simulink library "sm_trackV_lib_belt_contact_internal_sets"  (R2026a)
settings: Solver=VariableStepAuto
undefined symbols (not defined in the file): A, B, L01, L02, L03, L04, L05, L06, L07, L08, L09, L1, L10, L11, L12, L13, L14, L15, L16, L17, L18, L19, L2, L20, L21, L22, L23, L24, L25, L26, L27, L28, L29, L3, L30, L31, L32, L33, L34, L35, L36, L37, L38, L39, L40, L41, L42, L43, L44, L45, P00, P01, P02, P03, P04, P05, P06, P07, P08, P09 ... (+59)
libraries: sm_trackV_lib_belt_contact x132, $bdroot x51
Description:
  | Copyright 2024-2026 The MathWorks, Inc.
settings Model: Creator=smiller  LastModifiedBy=smiller

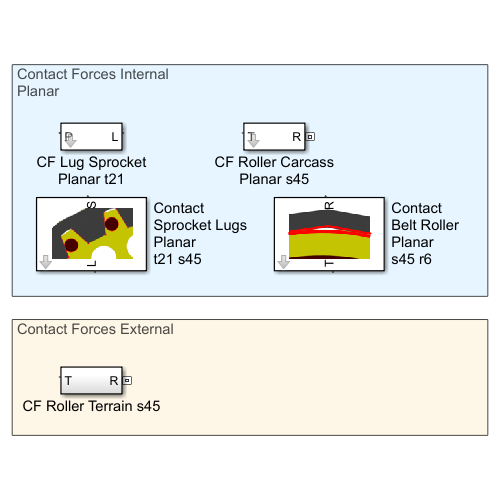
[thumbnail: Simulink's stored preview of the top-level diagram]
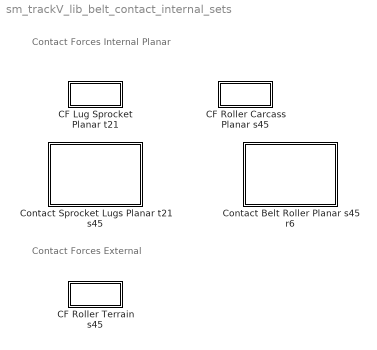
== system sm_trackV_lib_belt_contact_internal_sets ==
  note: Contact Forces External
  note: Contact Forces Internal
      | Planar
  CF Lug Sprocket Planar t21 : Subsystem  mask{K_SprocketLug=Trac.Contact.SprocketLug.K, B_SprocketLug=Trac.Contact.SprocketLug.B, TW_SprocketLug=Trac.Contact.SprocketLug.TW}
      mask prompts: K_SprocketLug "Normal Stiffness (N/m)"; B_SprocketLug "Normal Damping (N/(m/s))"; TW_SprocketLug "Normal Transition Width (m)"
  CF Roller Carcass Planar s45 : Subsystem  mask{K_Roller=Trac.Contact.Roller.K, B_Roller=Trac.Contact.Roller.B, TW_Roller=Trac.Contact.Roller.TW}
      mask prompts: K_Roller "Normal Stiffness (N/m)"; B_Roller "Normal Damping (N/(m/s))"; TW_Roller "Normal Transition Width (m)"
  CF Roller Terrain s45 : Subsystem
  Contact Belt Roller Planar s45 r6 : Subsystem  mask(Contact Force (Planar), Belt to 6 Rollers){K_SprocketRoller=Trac.Contact.SprocketRoller.K, B_SprocketRoller=Trac.Contact.SprocketRoller.B, TW_SprocketRoller=Trac.Contact.SprocketRoller.TW, K_IdlerFix=Trac.Contact.IdlerR.K, B_IdlerFix=Trac.Contact.IdlerR.B, TW_IdlerFix=Trac.Contact.IdlerR.TW, K_IdlerArm=Trac.Contact.IdlerF.K, B_IdlerArm=Trac.Contact.IdlerF.B, TW_IdlerArm=Trac.Contact.IdlerF.TW, K_Roller=Trac.Contact.Roller.K, B_Roller=Trac.Contact.Roller.B, TW_Roller=Trac.Contact.Roller.TW}
      mask prompts: K_SprocketRoller "Normal Stiffness (N/m)"; B_SprocketRoller "Normal Damping (N/(m/s))"; TW_SprocketRoller "Normal Transition Width (m)"; K_IdlerFix "Normal Stiffness (N/m)"; B_IdlerFix "Normal Damping (N/(m/s))"; TW_IdlerFix "Normal Transition Width (m)"; K_IdlerArm "Normal Stiffness (N/m)"; B_IdlerArm "Normal Damping (N/(m/s))"; TW_IdlerArm "Normal Transition Width (m)"; K_Roller "Normal Stiffness (N/m)"; B_Roller "Normal Damping (N/(m/s))"; TW_Roller "Normal Transition Width (m)"
      mask help: Models contact forces between entire belt (45 segments) and 6 rollers.
      mask TypeOptions K_SprocketRoller:
      | CF Roller
      | Sprocket/K_Roller
      mask TypeOptions B_SprocketRoller:
      | CF Roller
      | Sprocket/B_Roller
      mask TypeOptions TW_SprocketRoller:
      | CF Roller
      | Sprocket/TW_Roller
      mask TypeOptions K_IdlerFix:
      | CF Roller
      | Idler Fix/K_Roller
      mask TypeOptions B_IdlerFix:
      | CF Roller
      | Idler Fix/B_Roller
      mask TypeOptions TW_IdlerFix:
      | CF Roller
      | Idler Fix/TW_Roller
      mask TypeOptions K_IdlerArm:
      | CF Roller
      | Idler Arm/K_Roller
      mask TypeOptions B_IdlerArm:
      | CF Roller
      | Idler Arm/B_Roller
      mask TypeOptions TW_IdlerArm:
      | CF Roller
      | Idler Arm/TW_Roller
      mask TypeOptions K_Roller:
      | CF Roller
      | Roller L1/K_Roller | CF Roller
      | Roller L2/K_Roller | CF Roller
      | Roller L3/K_Roller
      mask TypeOptions B_Roller:
      | CF Roller
      | Roller L1/B_Roller | CF Roller
      | Roller L2/B_Roller | CF Roller
      | Roller L3/B_Roller
      mask TypeOptions TW_Roller:
      | CF Roller
      | Roller L1/TW_Roller | CF Roller
      | Roller L2/TW_Roller | CF Roller
      | Roller L3/TW_Roller
      mask DialogControl cont_contact_sprocketLug Prompt: Sprocket Roller
      mask DialogControl cont_contact_idlerFix Prompt: Idler Fixed
      mask DialogControl cont_contact_idlerArm Prompt: Idler Arm
      mask DialogControl cont_contact_rollerL Prompt: Lower Roller
      mask Display: image('sm_belt_cf_roller_carcass_IMAGE.png')
  Contact Sprocket Lugs Planar t21 s45 : Subsystem  mask(Contact Force (Planar), Belt to Sprocket){K_SprocketLug=Trac.Contact.SprocketLug.K, B_SprocketLug=Trac.Contact.SprocketLug.B, TW_SprocketLug=Trac.Contact.SprocketLug.TW}
      mask prompts: K_SprocketLug "Normal Stiffness (N/m)"; B_SprocketLug "Normal Damping (N/(m/s))"; TW_SprocketLug "Normal Transition Width (m)"
      mask help: Models contact forces between belt (45 lugs) and sprocket (21 pins).
      mask Display: image('sm_belt_cf_sprocket_lugs_IMAGE.png');

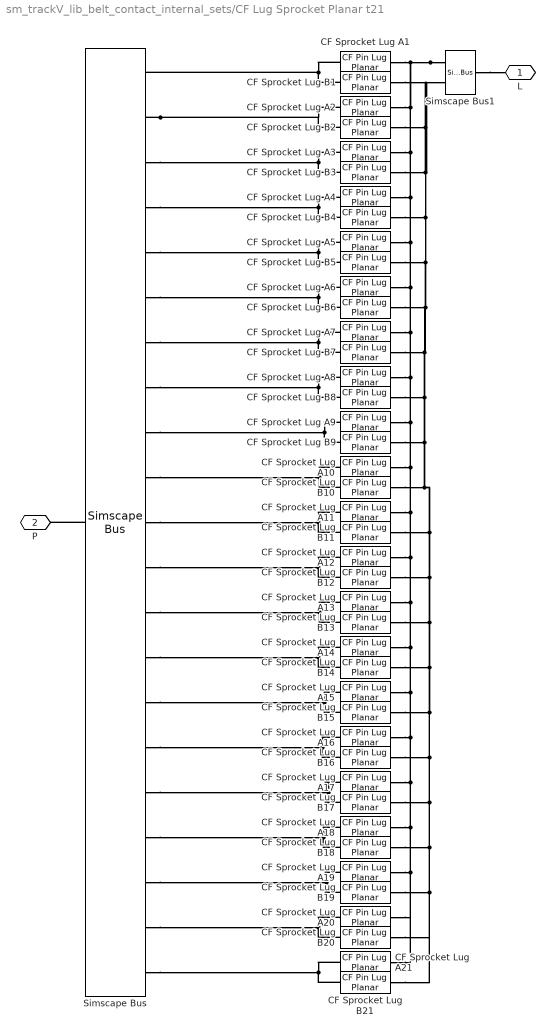
== system sm_trackV_lib_belt_contact_internal_sets/CF Lug Sprocket Planar t21 ==
  CF Sprocket Lug A{1..21} (21 alike) : sm_trackV_lib_belt_contact/CF Pin Lug Planar  K_SprocketLug=K_SprocketLug  B_SprocketLug=B_SprocketLug  TW_SprocketLug=TW_SprocketLug
  CF Sprocket Lug B{1..21} (21 alike) : sm_trackV_lib_belt_contact/CF Pin Lug Planar  K_SprocketLug=K_SprocketLug  B_SprocketLug=B_SprocketLug  TW_SprocketLug=TW_SprocketLug
  Simscape Bus : SimscapeBus  HierarchyStrings=P00;P01;P02;P03;P04;P05;P06;P07;P08;P09;P10;P11;P12;P13;P14;P15;P16;P17;P18;P19;P20
  Simscape Bus1 : SimscapeBus  HierarchyStrings=A;B  ConnectionType=Bus: CBO_TreadLug
  L : PMIOPort  Side=Right
  P : PMIOPort  Port=2  Side=Left
  connections:
  Simscape Bus/LConn4 -- CF Sprocket Lug B4/LConn1 -- CF Sprocket Lug A4/LConn1
  Simscape Bus/LConn13 -- CF Sprocket Lug B13/LConn1 -- CF Sprocket Lug A13/LConn1
  Simscape Bus/LConn12 -- CF Sprocket Lug B12/LConn1 -- CF Sprocket Lug A12/LConn1
  Simscape Bus/LConn3 -- CF Sprocket Lug B3/LConn1 -- CF Sprocket Lug A3/LConn1
  Simscape Bus/LConn15 -- CF Sprocket Lug B15/LConn1 -- CF Sprocket Lug A15/LConn1
  Simscape Bus/LConn17 -- CF Sprocket Lug B17/LConn1 -- CF Sprocket Lug A17/LConn1
  Simscape Bus/LConn14 -- CF Sprocket Lug B14/LConn1 -- CF Sprocket Lug A14/LConn1
  Simscape Bus/LConn8 -- CF Sprocket Lug A8/LConn1 -- CF Sprocket Lug B8/LConn1
  Simscape Bus1/LConn1 -- CF Sprocket Lug A1/RConn1 -- CF Sprocket Lug A2/RConn1 -- CF Sprocket Lug A3/RConn1 -- CF Sprocket Lug A4/RConn1 -- CF Sprocket Lug A5/RConn1 -- CF Sprocket Lug A6/RConn1 -- CF Sprocket Lug A7/RConn1 -- CF Sprocket Lug A8/RConn1 -- CF Sprocket Lug A9/RConn1 -- CF Sprocket Lug A10/RConn1 -- CF Sprocket Lug A11/RConn1 -- CF Sprocket Lug A12/RConn1 -- CF Sprocket Lug A13/RConn1 -- CF Sprocket Lug A14/RConn1 -- CF Sprocket Lug A15/RConn1 -- CF Sprocket Lug A16/RConn1 -- CF Sprocket Lug A17/RConn1 -- CF Sprocket Lug A18/RConn1 -- CF Sprocket Lug A19/RConn1 -- CF Sprocket Lug A21/RConn1 -- CF Sprocket Lug A20/RConn1
  Simscape Bus/LConn21 -- CF Sprocket Lug A21/LConn1 -- CF Sprocket Lug B21/LConn1
  CF Sprocket Lug B17/RConn1 -- CF Sprocket Lug B18/RConn1 -- CF Sprocket Lug B19/RConn1 -- CF Sprocket Lug B21/RConn1 -- CF Sprocket Lug B20/RConn1 -- CF Sprocket Lug B16/RConn1 -- CF Sprocket Lug B15/RConn1 -- CF Sprocket Lug B14/RConn1 -- CF Sprocket Lug B13/RConn1 -- CF Sprocket Lug B12/RConn1 -- CF Sprocket Lug B11/RConn1 -- CF Sprocket Lug B10/RConn1 -- CF Sprocket Lug B9/RConn1 -- CF Sprocket Lug B8/RConn1 -- CF Sprocket Lug B7/RConn1 -- CF Sprocket Lug B6/RConn1 -- CF Sprocket Lug B5/RConn1 -- CF Sprocket Lug B4/RConn1 -- CF Sprocket Lug B3/RConn1 -- CF Sprocket Lug B2/RConn1 -- CF Sprocket Lug B1/RConn1 -- Simscape Bus1/LConn2
  Simscape Bus/LConn19 -- CF Sprocket Lug B19/LConn1 -- CF Sprocket Lug A19/LConn1
  Simscape Bus/LConn16 -- CF Sprocket Lug B16/LConn1 -- CF Sprocket Lug A16/LConn1
  Simscape Bus/LConn9 -- CF Sprocket Lug A9/LConn1 -- CF Sprocket Lug B9/LConn1
  Simscape Bus/LConn7 -- CF Sprocket Lug A7/LConn1 -- CF Sprocket Lug B7/LConn1
  CF Sprocket Lug A1/LConn1 -- CF Sprocket Lug B1/LConn1 -- Simscape Bus/LConn1
  Simscape Bus/LConn6 -- CF Sprocket Lug B6/LConn1 -- CF Sprocket Lug A6/LConn1
  Simscape Bus/LConn10 -- CF Sprocket Lug B10/LConn1 -- CF Sprocket Lug A10/LConn1
  Simscape Bus/LConn11 -- CF Sprocket Lug A11/LConn1 -- CF Sprocket Lug B11/LConn1
  Simscape Bus/LConn2 -- CF Sprocket Lug A2/LConn1 -- CF Sprocket Lug B2/LConn1
  Simscape Bus/LConn18 -- CF Sprocket Lug B18/LConn1 -- CF Sprocket Lug A18/LConn1
  Simscape Bus/LConn5 -- CF Sprocket Lug B5/LConn1 -- CF Sprocket Lug A5/LConn1
  Simscape Bus/LConn20 -- CF Sprocket Lug B20/LConn1 -- CF Sprocket Lug A20/LConn1
  Simscape Bus/RConn1 -- P/RConn1
  Simscape Bus1/RConn1 -- L/RConn1

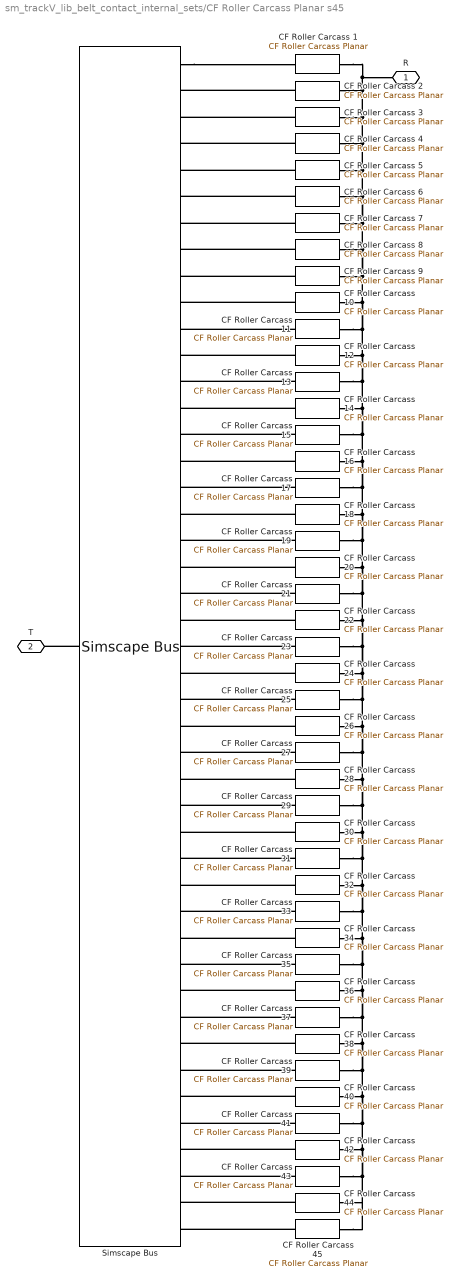
== system sm_trackV_lib_belt_contact_internal_sets/CF Roller Carcass Planar s45 ==
  CF Roller Carcass {1..45} (45 alike) : sm_trackV_lib_belt_contact/CF Roller Carcass Planar  K_Roller=K_Roller  B_Roller=B_Roller  TW_Roller=TW_Roller
  Simscape Bus : SimscapeBus  HierarchyStrings=T01;T02;T03;T04;T05;T06;T07;T08;T09;T10;T11;T12;T13;T14;T15;T16;T17;T18;T19;T20;T21;T22;T23;T24;T25;T26;T27;T28;T29;T30;T31;T32;T33;T34;T35;T36;T37;T38;T39;T40;T41;T42;T43;T44;T45  ConnectionType=Bus: CBO_TrRoll
  R : PMIOPort  Side=Left
  T : PMIOPort  Port=2  Side=Right
  connections:
  Simscape Bus/RConn1 -- T/RConn1
  Simscape Bus/LConn1 -- CF Roller Carcass 1/LConn1
  CF Roller Carcass 2/LConn1 -- Simscape Bus/LConn2
  CF Roller Carcass 5/RConn1 -- CF Roller Carcass 6/RConn1 -- CF Roller Carcass 7/RConn1 -- CF Roller Carcass 8/RConn1 -- CF Roller Carcass 9/RConn1 -- CF Roller Carcass 10/RConn1 -- CF Roller Carcass 11/RConn1 -- CF Roller Carcass 12/RConn1 -- CF Roller Carcass 13/RConn1 -- CF Roller Carcass 14/RConn1 -- CF Roller Carcass 15/RConn1 -- CF Roller Carcass 16/RConn1 -- CF Roller Carcass 17/RConn1 -- CF Roller Carcass 18/RConn1 -- CF Roller Carcass 19/RConn1 -- CF Roller Carcass 20/RConn1 -- CF Roller Carcass 21/RConn1 -- CF Roller Carcass 22/RConn1 -- CF Roller Carcass 23/RConn1 -- CF Roller Carcass 24/RConn1 -- CF Roller Carcass 25/RConn1 -- CF Roller Carcass 26/RConn1 -- CF Roller Carcass 27/RConn1 -- CF Roller Carcass 28/RConn1 -- CF Roller Carcass 29/RConn1 -- CF Roller Carcass 30/RConn1 -- CF Roller Carcass 31/RConn1 -- CF Roller Carcass 32/RConn1 -- CF Roller Carcass 33/RConn1 -- CF Roller Carcass 34/RConn1 -- CF Roller Carcass 35/RConn1 -- CF Roller Carcass 36/RConn1 -- CF Roller Carcass 37/RConn1 -- CF Roller Carcass 38/RConn1 -- CF Roller Carcass 39/RConn1 -- CF Roller Carcass 40/RConn1 -- CF Roller Carcass 41/RConn1 -- CF Roller Carcass 42/RConn1 -- CF Roller Carcass 43/RConn1 -- CF Roller Carcass 45/RConn1 -- CF Roller Carcass 44/RConn1 -- CF Roller Carcass 4/RConn1 -- CF Roller Carcass 3/RConn1 -- CF Roller Carcass 2/RConn1 -- CF Roller Carcass 1/RConn1 -- R/RConn1
  CF Roller Carcass 3/LConn1 -- Simscape Bus/LConn3
  CF Roller Carcass 4/LConn1 -- Simscape Bus/LConn4
  CF Roller Carcass 5/LConn1 -- Simscape Bus/LConn5
  CF Roller Carcass 9/LConn1 -- Simscape Bus/LConn9
  CF Roller Carcass 8/LConn1 -- Simscape Bus/LConn8
  CF Roller Carcass 10/LConn1 -- Simscape Bus/LConn10
  CF Roller Carcass 7/LConn1 -- Simscape Bus/LConn7
  CF Roller Carcass 6/LConn1 -- Simscape Bus/LConn6
  CF Roller Carcass 14/LConn1 -- Simscape Bus/LConn14
  CF Roller Carcass 13/LConn1 -- Simscape Bus/LConn13
  CF Roller Carcass 15/LConn1 -- Simscape Bus/LConn15
  CF Roller Carcass 12/LConn1 -- Simscape Bus/LConn12
  CF Roller Carcass 11/LConn1 -- Simscape Bus/LConn11
  CF Roller Carcass 18/LConn1 -- Simscape Bus/LConn18
  CF Roller Carcass 21/LConn1 -- Simscape Bus/LConn21
  CF Roller Carcass 17/LConn1 -- Simscape Bus/LConn17
  CF Roller Carcass 22/LConn1 -- Simscape Bus/LConn22
  CF Roller Carcass 23/LConn1 -- Simscape Bus/LConn23
  CF Roller Carcass 16/LConn1 -- Simscape Bus/LConn16
  CF Roller Carcass 24/LConn1 -- Simscape Bus/LConn24
  CF Roller Carcass 19/LConn1 -- Simscape Bus/LConn19
  CF Roller Carcass 25/LConn1 -- Simscape Bus/LConn25
  CF Roller Carcass 20/LConn1 -- Simscape Bus/LConn20
  CF Roller Carcass 26/LConn1 -- Simscape Bus/LConn26
  CF Roller Carcass 30/LConn1 -- Simscape Bus/LConn30
  CF Roller Carcass 29/LConn1 -- Simscape Bus/LConn29
  CF Roller Carcass 28/LConn1 -- Simscape Bus/LConn28
  CF Roller Carcass 27/LConn1 -- Simscape Bus/LConn27
  CF Roller Carcass 31/LConn1 -- Simscape Bus/LConn31
  CF Roller Carcass 34/LConn1 -- Simscape Bus/LConn34
  CF Roller Carcass 35/LConn1 -- Simscape Bus/LConn35
  CF Roller Carcass 36/LConn1 -- Simscape Bus/LConn36
  CF Roller Carcass 33/LConn1 -- Simscape Bus/LConn33
  CF Roller Carcass 32/LConn1 -- Simscape Bus/LConn32
  CF Roller Carcass 37/LConn1 -- Simscape Bus/LConn37
  CF Roller Carcass 39/LConn1 -- Simscape Bus/LConn39
  CF Roller Carcass 42/LConn1 -- Simscape Bus/LConn42
  CF Roller Carcass 41/LConn1 -- Simscape Bus/LConn41
  CF Roller Carcass 40/LConn1 -- Simscape Bus/LConn40
  CF Roller Carcass 38/LConn1 -- Simscape Bus/LConn38
  CF Roller Carcass 43/LConn1 -- Simscape Bus/LConn43
  CF Roller Carcass 44/LConn1 -- Simscape Bus/LConn44
  CF Roller Carcass 45/LConn1 -- Simscape Bus/LConn45

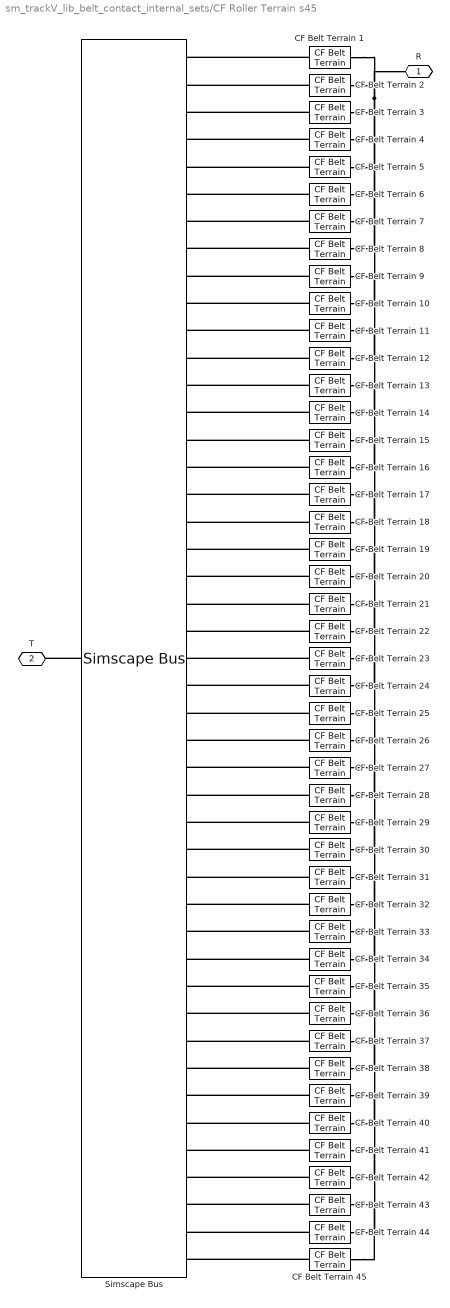
== system sm_trackV_lib_belt_contact_internal_sets/CF Roller Terrain s45 ==
  CF Belt Terrain {1..45} (45 alike) : sm_trackV_lib_belt_contact/CF Belt Terrain  NormalStiffness=Scene.Contact.Terrain.K  NormalDamping=Scene.Contact.Terrain.B  NormalTransitionRegionWidth=Scene.Contact.Terrain.TW  CoefficientOfDynamicFriction=Scene.Contact.Terrain.mud  CoefficientOfStaticFriction=Scene.Contact.Terrain.mus  FrictionalCriticalVelocity=Scene.Contact.Terrain.CV
  Simscape Bus : SimscapeBus  HierarchyStrings=T01;T02;T03;T04;T05;T06;T07;T08;T09;T10;T11;T12;T13;T14;T15;T16;T17;T18;T19;T20;T21;T22;T23;T24;T25;T26;T27;T28;T29;T30;T31;T32;T33;T34;T35;T36;T37;T38;T39;T40;T41;T42;T43;T44;T45  ConnectionType=Bus: CBO_TrRoll
  R : PMIOPort  Side=Left
  T : PMIOPort  Port=2  Side=Right
  connections:
  CF Belt Terrain 45/LConn1 -- Simscape Bus/LConn45
  CF Belt Terrain 44/LConn1 -- Simscape Bus/LConn44
  CF Belt Terrain 43/LConn1 -- Simscape Bus/LConn43
  CF Belt Terrain 38/LConn1 -- Simscape Bus/LConn38
  CF Belt Terrain 40/LConn1 -- Simscape Bus/LConn40
  CF Belt Terrain 41/LConn1 -- Simscape Bus/LConn41
  CF Belt Terrain 42/LConn1 -- Simscape Bus/LConn42
  CF Belt Terrain 39/LConn1 -- Simscape Bus/LConn39
  CF Belt Terrain 37/LConn1 -- Simscape Bus/LConn37
  CF Belt Terrain 32/LConn1 -- Simscape Bus/LConn32
  CF Belt Terrain 33/LConn1 -- Simscape Bus/LConn33
  CF Belt Terrain 36/LConn1 -- Simscape Bus/LConn36
  CF Belt Terrain 35/LConn1 -- Simscape Bus/LConn35
  CF Belt Terrain 34/LConn1 -- Simscape Bus/LConn34
  CF Belt Terrain 31/LConn1 -- Simscape Bus/LConn31
  CF Belt Terrain 27/LConn1 -- Simscape Bus/LConn27
  CF Belt Terrain 28/LConn1 -- Simscape Bus/LConn28
  CF Belt Terrain 29/LConn1 -- Simscape Bus/LConn29
  CF Belt Terrain 30/LConn1 -- Simscape Bus/LConn30
  CF Belt Terrain 26/LConn1 -- Simscape Bus/LConn26
  CF Belt Terrain 20/LConn1 -- Simscape Bus/LConn20
  CF Belt Terrain 25/LConn1 -- Simscape Bus/LConn25
  CF Belt Terrain 19/LConn1 -- Simscape Bus/LConn19
  CF Belt Terrain 24/LConn1 -- Simscape Bus/LConn24
  CF Belt Terrain 16/LConn1 -- Simscape Bus/LConn16
  CF Belt Terrain 23/LConn1 -- Simscape Bus/LConn23
  CF Belt Terrain 22/LConn1 -- Simscape Bus/LConn22
  CF Belt Terrain 17/LConn1 -- Simscape Bus/LConn17
  CF Belt Terrain 21/LConn1 -- Simscape Bus/LConn21
  CF Belt Terrain 18/LConn1 -- Simscape Bus/LConn18
  CF Belt Terrain 11/LConn1 -- Simscape Bus/LConn11
  CF Belt Terrain 12/LConn1 -- Simscape Bus/LConn12
  CF Belt Terrain 15/LConn1 -- Simscape Bus/LConn15
  CF Belt Terrain 13/LConn1 -- Simscape Bus/LConn13
  CF Belt Terrain 14/LConn1 -- Simscape Bus/LConn14
  CF Belt Terrain 6/LConn1 -- Simscape Bus/LConn6
  CF Belt Terrain 7/LConn1 -- Simscape Bus/LConn7
  CF Belt Terrain 10/LConn1 -- Simscape Bus/LConn10
  CF Belt Terrain 8/LConn1 -- Simscape Bus/LConn8
  CF Belt Terrain 9/LConn1 -- Simscape Bus/LConn9
  CF Belt Terrain 5/LConn1 -- Simscape Bus/LConn5
  CF Belt Terrain 4/LConn1 -- Simscape Bus/LConn4
  CF Belt Terrain 3/LConn1 -- Simscape Bus/LConn3
  CF Belt Terrain 44/RConn1 -- CF Belt Terrain 43/RConn1 -- CF Belt Terrain 42/RConn1 -- CF Belt Terrain 41/RConn1 -- CF Belt Terrain 40/RConn1 -- CF Belt Terrain 39/RConn1 -- CF Belt Terrain 38/RConn1 -- CF Belt Terrain 37/RConn1 -- CF Belt Terrain 36/RConn1 -- CF Belt Terrain 35/RConn1 -- CF Belt Terrain 34/RConn1 -- CF Belt Terrain 33/RConn1 -- CF Belt Terrain 32/RConn1 -- CF Belt Terrain 31/RConn1 -- CF Belt Terrain 30/RConn1 -- CF Belt Terrain 29/RConn1 -- CF Belt Terrain 28/RConn1 -- CF Belt Terrain 27/RConn1 -- CF Belt Terrain 26/RConn1 -- CF Belt Terrain 25/RConn1 -- CF Belt Terrain 24/RConn1 -- CF Belt Terrain 23/RConn1 -- CF Belt Terrain 22/RConn1 -- CF Belt Terrain 21/RConn1 -- CF Belt Terrain 20/RConn1 -- CF Belt Terrain 19/RConn1 -- CF Belt Terrain 18/RConn1 -- CF Belt Terrain 17/RConn1 -- CF Belt Terrain 16/RConn1 -- CF Belt Terrain 15/RConn1 -- CF Belt Terrain 14/RConn1 -- CF Belt Terrain 13/RConn1 -- CF Belt Terrain 12/RConn1 -- CF Belt Terrain 11/RConn1 -- CF Belt Terrain 10/RConn1 -- CF Belt Terrain 9/RConn1 -- CF Belt Terrain 8/RConn1 -- CF Belt Terrain 7/RConn1 -- CF Belt Terrain 6/RConn1 -- CF Belt Terrain 5/RConn1 -- CF Belt Terrain 4/RConn1 -- CF Belt Terrain 3/RConn1 -- CF Belt Terrain 2/RConn1 -- CF Belt Terrain 1/RConn1 -- R/RConn1 -- CF Belt Terrain 45/RConn1
  CF Belt Terrain 2/LConn1 -- Simscape Bus/LConn2
  CF Belt Terrain 1/LConn1 -- Simscape Bus/LConn1
  Simscape Bus/RConn1 -- T/RConn1

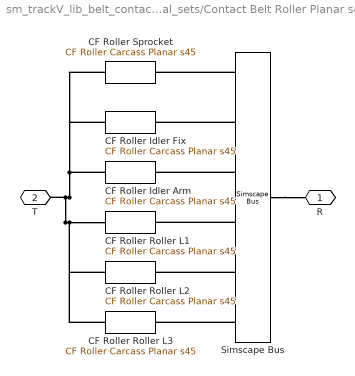
== system sm_trackV_lib_belt_contact_internal_sets/Contact Belt Roller Planar s45 r6 ==
  CF Roller Idler Arm : $bdroot/CF Roller Carcass Planar s45  K_Roller=K_IdlerArm  B_Roller=B_IdlerArm  TW_Roller=TW_IdlerArm
  CF Roller Idler Fix : $bdroot/CF Roller Carcass Planar s45  K_Roller=K_IdlerFix  B_Roller=B_IdlerFix  TW_Roller=TW_IdlerFix
  CF Roller Roller L1 : $bdroot/CF Roller Carcass Planar s45  K_Roller=K_Roller  B_Roller=B_Roller  TW_Roller=TW_Roller
  CF Roller Roller L2 : $bdroot/CF Roller Carcass Planar s45  K_Roller=K_Roller  B_Roller=B_Roller  TW_Roller=TW_Roller
  CF Roller Roller L3 : $bdroot/CF Roller Carcass Planar s45  K_Roller=K_Roller  B_Roller=B_Roller  TW_Roller=TW_Roller
  CF Roller Sprocket : $bdroot/CF Roller Carcass Planar s45  K_Roller=K_SprocketRoller  B_Roller=B_SprocketRoller  TW_Roller=TW_SprocketRoller
  Simscape Bus : SimscapeBus  HierarchyStrings=S;X;A;L1;L2;L3
  R : PMIOPort  Side=Right
  T : PMIOPort  Port=2  Side=Left
  connections:
  T/RConn1 -- CF Roller Idler Arm/RConn1 -- CF Roller Sprocket/RConn1 -- CF Roller Idler Fix/RConn1 -- CF Roller Roller L3/RConn1 -- CF Roller Roller L2/RConn1 -- CF Roller Roller L1/RConn1
  Simscape Bus/LConn2 -- CF Roller Idler Fix/LConn1
  Simscape Bus/RConn1 -- R/RConn1
  Simscape Bus/LConn1 -- CF Roller Sprocket/LConn1
  Simscape Bus/LConn3 -- CF Roller Idler Arm/LConn1
  Simscape Bus/LConn4 -- CF Roller Roller L1/LConn1
  Simscape Bus/LConn5 -- CF Roller Roller L2/LConn1
  Simscape Bus/LConn6 -- CF Roller Roller L3/LConn1

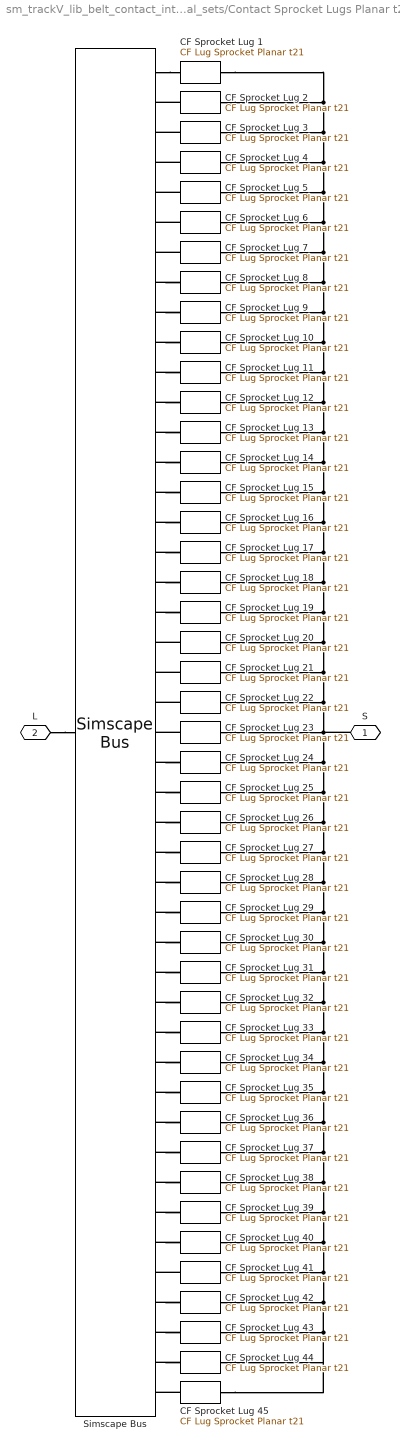
== system sm_trackV_lib_belt_contact_internal_sets/Contact Sprocket Lugs Planar t21 s45 ==
  CF Sprocket Lug {1..45} (45 alike) : $bdroot/CF Lug Sprocket Planar t21  K_SprocketLug=K_SprocketLug  B_SprocketLug=B_SprocketLug  TW_SprocketLug=TW_SprocketLug
  Simscape Bus : SimscapeBus  HierarchyStrings=L01;L02;L03;L04;L05;L06;L07;L08;L09;L10;L11;L12;L13;L14;L15;L16;L17;L18;L19;L20;L21;L22;L23;L24;L25;L26;L27;L28;L29;L30;L31;L32;L33;L34;L35;L36;L37;L38;L39;L40;L41;L42;L43;L44;L45  ConnectionType=Bus: CBO_TrSpr
  S : PMIOPort  Side=Left
  L : PMIOPort  Port=2  Side=Right
  connections:
  CF Sprocket Lug 1/LConn1 -- CF Sprocket Lug 3/LConn1 -- CF Sprocket Lug 4/LConn1 -- CF Sprocket Lug 5/LConn1 -- CF Sprocket Lug 6/LConn1 -- CF Sprocket Lug 7/LConn1 -- CF Sprocket Lug 8/LConn1 -- CF Sprocket Lug 9/LConn1 -- CF Sprocket Lug 10/LConn1 -- CF Sprocket Lug 11/LConn1 -- CF Sprocket Lug 12/LConn1 -- CF Sprocket Lug 13/LConn1 -- CF Sprocket Lug 14/LConn1 -- CF Sprocket Lug 15/LConn1 -- CF Sprocket Lug 16/LConn1 -- CF Sprocket Lug 17/LConn1 -- CF Sprocket Lug 18/LConn1 -- CF Sprocket Lug 19/LConn1 -- CF Sprocket Lug 20/LConn1 -- CF Sprocket Lug 21/LConn1 -- CF Sprocket Lug 22/LConn1 -- CF Sprocket Lug 23/LConn1 -- CF Sprocket Lug 24/LConn1 -- CF Sprocket Lug 25/LConn1 -- CF Sprocket Lug 26/LConn1 -- CF Sprocket Lug 27/LConn1 -- CF Sprocket Lug 28/LConn1 -- CF Sprocket Lug 29/LConn1 -- CF Sprocket Lug 30/LConn1 -- CF Sprocket Lug 31/LConn1 -- CF Sprocket Lug 32/LConn1 -- CF Sprocket Lug 33/LConn1 -- CF Sprocket Lug 34/LConn1 -- CF Sprocket Lug 35/LConn1 -- CF Sprocket Lug 36/LConn1 -- CF Sprocket Lug 37/LConn1 -- CF Sprocket Lug 38/LConn1 -- CF Sprocket Lug 39/LConn1 -- CF Sprocket Lug 40/LConn1 -- CF Sprocket Lug 41/LConn1 -- CF Sprocket Lug 42/LConn1 -- CF Sprocket Lug 43/LConn1 -- CF Sprocket Lug 45/LConn1 -- CF Sprocket Lug 44/LConn1 -- S/RConn1 -- CF Sprocket Lug 2/LConn1
  L/RConn1 -- Simscape Bus/RConn1
  CF Sprocket Lug 2/RConn1 -- Simscape Bus/LConn2
  CF Sprocket Lug 4/RConn1 -- Simscape Bus/LConn4
  CF Sprocket Lug 3/RConn1 -- Simscape Bus/LConn3
  Simscape Bus/LConn1 -- CF Sprocket Lug 1/RConn1
  CF Sprocket Lug 5/RConn1 -- Simscape Bus/LConn5
  CF Sprocket Lug 7/RConn1 -- Simscape Bus/LConn7
  CF Sprocket Lug 8/RConn1 -- Simscape Bus/LConn8
  CF Sprocket Lug 6/RConn1 -- Simscape Bus/LConn6
  CF Sprocket Lug 13/RConn1 -- Simscape Bus/LConn13
  CF Sprocket Lug 16/RConn1 -- Simscape Bus/LConn16
  CF Sprocket Lug 14/RConn1 -- Simscape Bus/LConn14
  CF Sprocket Lug 9/RConn1 -- Simscape Bus/LConn9
  CF Sprocket Lug 11/RConn1 -- Simscape Bus/LConn11
  CF Sprocket Lug 12/RConn1 -- Simscape Bus/LConn12
  CF Sprocket Lug 10/RConn1 -- Simscape Bus/LConn10
  CF Sprocket Lug 15/RConn1 -- Simscape Bus/LConn15
  CF Sprocket Lug 31/RConn1 -- Simscape Bus/LConn31
  CF Sprocket Lug 26/RConn1 -- Simscape Bus/LConn26
  CF Sprocket Lug 28/RConn1 -- Simscape Bus/LConn28
  CF Sprocket Lug 27/RConn1 -- Simscape Bus/LConn27
  CF Sprocket Lug 30/RConn1 -- Simscape Bus/LConn30
  CF Sprocket Lug 32/RConn1 -- Simscape Bus/LConn32
  CF Sprocket Lug 29/RConn1 -- Simscape Bus/LConn29
  CF Sprocket Lug 21/RConn1 -- Simscape Bus/LConn21
  CF Sprocket Lug 25/RConn1 -- Simscape Bus/LConn25
  CF Sprocket Lug 24/RConn1 -- Simscape Bus/LConn24
  CF Sprocket Lug 22/RConn1 -- Simscape Bus/LConn22
  CF Sprocket Lug 17/RConn1 -- Simscape Bus/LConn17
  CF Sprocket Lug 19/RConn1 -- Simscape Bus/LConn19
  CF Sprocket Lug 20/RConn1 -- Simscape Bus/LConn20
  CF Sprocket Lug 18/RConn1 -- Simscape Bus/LConn18
  CF Sprocket Lug 23/RConn1 -- Simscape Bus/LConn23
  CF Sprocket Lug 33/RConn1 -- Simscape Bus/LConn33
  CF Sprocket Lug 38/RConn1 -- Simscape Bus/LConn38
  CF Sprocket Lug 37/RConn1 -- Simscape Bus/LConn37
  CF Sprocket Lug 35/RConn1 -- Simscape Bus/LConn35
  CF Sprocket Lug 36/RConn1 -- Simscape Bus/LConn36
  CF Sprocket Lug 40/RConn1 -- Simscape Bus/LConn40
  CF Sprocket Lug 34/RConn1 -- Simscape Bus/LConn34
  CF Sprocket Lug 39/RConn1 -- Simscape Bus/LConn39
  CF Sprocket Lug 44/RConn1 -- Simscape Bus/LConn44
  CF Sprocket Lug 45/RConn1 -- Simscape Bus/LConn45
  CF Sprocket Lug 41/RConn1 -- Simscape Bus/LConn41
  CF Sprocket Lug 42/RConn1 -- Simscape Bus/LConn42
  CF Sprocket Lug 43/RConn1 -- Simscape Bus/LConn43
